simulink model "APP_SelSig1"  (R2016b)
settings: configuration reference "CodeGenConfigSet" (kept outside this file)
values from neighbouring files (symbols this model uses):
  APP_duLimErrPos_C = Calibration.Parameter    [init_APP_SelSig.m]
  APP_uAPPDef_C = Calibration.Parameter    [init_APP_SelSig.m]
  APP_uRaw2Offset_C = Calibration.Parameter    [init_APP_SelSig.m]
  MoFAPP_dRawSigFac_C = Calibration.Parameter    [init_APP_SelSig.m]
undefined symbols (not defined in the file or in its folder): APP_SelSig_DT
libraries: CXLib x3
settings Model: Creator=lenovo  LastModifiedBy=bianxuyin
settings ConfigSetRef: SourceLocation=Base Workspace

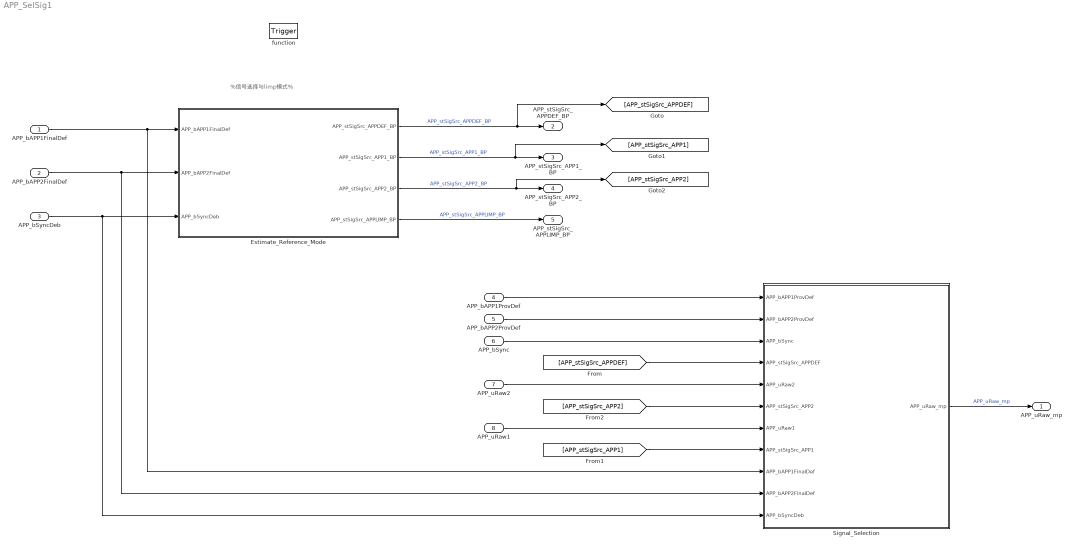
== system APP_SelSig1 ==
  note: %信号选择与limp模式%
  APP_bAPP1FinalDef : Inport  Description=Status Sensor 1 of the acceleration pedal finally defect  OutMin=0  OutMax=1  OutDataTypeStr=boolean
  APP_bAPP2FinalDef : Inport  Description=Status Sensor 2 of the acceleration pedal finally defect  Port=2  OutMin=0  OutMax=1  OutDataTypeStr=boolean
  APP_bSyncDeb : Inport  Description=Status debounced sync check  Port=3  OutMin=0  OutMax=1  OutDataTypeStr=boolean
  APP_bAPP1ProvDef : Inport  Description=Status Sensor 1 of the acceleration pedal temporary defect  Port=4  OutMin=0  OutMax=1  OutDataTypeStr=boolean
  APP_bAPP2ProvDef : Inport  Description=Status Sensor 2 of the acceleration pedal temporary defect  Port=5  OutMin=0  OutMax=1  OutDataTypeStr=boolean
  APP_bSync : Inport  Description=Status temporary sync check  Port=6  OutMin=0  OutMax=1  OutDataTypeStr=boolean
  APP_uRaw2 : Inport  Tag=mv  Description=Acceleration Pedal Position E  Port=7  OutMin=0  OutMax=5000  OutDataTypeStr=Ad_mv
  APP_uRaw1 : Inport  Tag=mv  Description=Acceleration Pedal Position D  Port=8  OutMin=0  OutMax=5000  OutDataTypeStr=Ad_mv
  function : TriggerPort  TriggerType=function-call  VariantControl=Variant
  Estimate_Reference_Mode : Subsystem
  Signal_Selection : Subsystem
  APP_uRaw_mp : Outport  Tag=mv  Description=Acceleration pedal position raw value  OutMin=0  OutMax=5000  OutDataTypeStr=Ad_mv
  APP_stSigSrc_APPDEF_BP : Outport  Description=both the sensors are defective. Use the default value  Port=2  OutMin=0  OutMax=1  OutDataTypeStr=boolean
  APP_stSigSrc_APP1_BP : Outport  Description=Sensor 1 is the reference variable, Sensor 2 value is defective  Port=3  OutMin=0  OutMax=1  OutDataTypeStr=boolean
  APP_stSigSrc_APP2_BP : Outport  Description=Sensor 2 is the reference variable,Sensor1 value is defective  Port=4  OutMin=0  OutMax=1  OutDataTypeStr=boolean
  APP_stSigSrc_APPLIMP_BP : Outport  Description=Substitute operation active, accelerator pedal sensor value and accelerator pedal sensor increase are limited  Port=5  OutMin=0  OutMax=1  OutDataTypeStr=boolean
  wires:
  Estimate_Reference_Mode/4(APP_stSigSrc_APPLIMP_BP) -> APP_stSigSrc_APPLIMP_BP/1  "APP_stSigSrc_APPLIMP_BP"
  Estimate_Reference_Mode/1(APP_stSigSrc_APPDEF_BP) -> [APP_stSigSrc_APPDEF], APP_stSigSrc_APPDEF_BP/1  "APP_stSigSrc_APPDEF_BP"
  Estimate_Reference_Mode/2(APP_stSigSrc_APP1_BP) -> [APP_stSigSrc_APP1], APP_stSigSrc_APP1_BP/1  "APP_stSigSrc_APP1_BP"
  Estimate_Reference_Mode/3(APP_stSigSrc_APP2_BP) -> APP_stSigSrc_APP2_BP/1, [APP_stSigSrc_APP2]  "APP_stSigSrc_APP2_BP"
  APP_bSyncDeb/1 -> Signal_Selection/11(APP_bSyncDeb), Estimate_Reference_Mode/3(APP_bSyncDeb)
  APP_bAPP2FinalDef/1 -> Signal_Selection/10(APP_bAPP2FinalDef), Estimate_Reference_Mode/2(APP_bAPP2FinalDef)
  APP_bAPP1FinalDef/1 -> Signal_Selection/9(APP_bAPP1FinalDef), Estimate_Reference_Mode/1(APP_bAPP1FinalDef)
  APP_bAPP1ProvDef/1 -> Signal_Selection/1(APP_bAPP1ProvDef)
  APP_bAPP2ProvDef/1 -> Signal_Selection/2(APP_bAPP2ProvDef)
  APP_bSync/1 -> Signal_Selection/3(APP_bSync)
  [APP_stSigSrc_APPDEF] -> Signal_Selection/4(APP_stSigSrc_APPDEF)
  APP_uRaw2/1 -> Signal_Selection/5(APP_uRaw2)
  [APP_stSigSrc_APP2] -> Signal_Selection/6(APP_stSigSrc_APP2)
  APP_uRaw1/1 -> Signal_Selection/7(APP_uRaw1)
  Signal_Selection/1(APP_uRaw_mp) -> APP_uRaw_mp/1  "APP_uRaw_mp"
  [APP_stSigSrc_APP1] -> Signal_Selection/8(APP_stSigSrc_APP1)

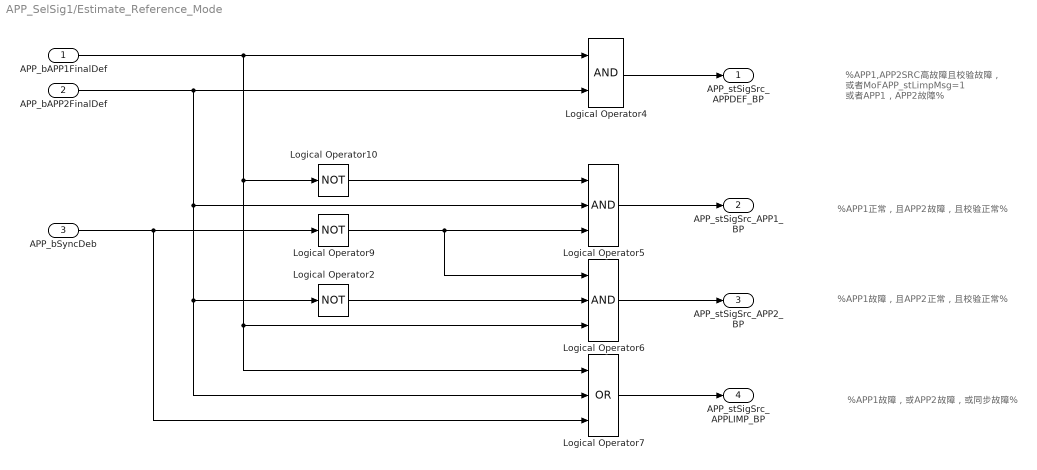
== system APP_SelSig1/Estimate_Reference_Mode ==
  note: %APP1正常，且APP2故障，且校验正常%
  note: %APP1故障，且APP2正常，且校验正常%
  note: %APP1故障，或APP2故障，或同步故障%
  note: %APP1,APP2SRC高故障且校验故障，
      | 或者MoFAPP_stLimpMsg=1
      | 或者APP1，APP2故障%
  APP_bAPP1FinalDef : Inport
  APP_bAPP2FinalDef : Inport  Port=2
  APP_bSyncDeb : Inport  Port=3
  Logical Operator10 : Logic  Operator=NOT  AllPortsSameDT=off  OutDataTypeStr=boolean
  Logical Operator2 : Logic  Operator=NOT  AllPortsSameDT=off  OutDataTypeStr=boolean
  Logical Operator4 : Logic  OutDataTypeStr=boolean
  Logical Operator5 : Logic  Inputs=3  OutDataTypeStr=boolean
  Logical Operator6 : Logic  Inputs=3  OutDataTypeStr=boolean
  Logical Operator7 : Logic  Operator=OR  Inputs=3  OutDataTypeStr=boolean
  Logical Operator9 : Logic  Operator=NOT  AllPortsSameDT=off  OutDataTypeStr=boolean
  APP_stSigSrc_APPDEF_BP : Outport
  APP_stSigSrc_APP1_BP : Outport  Port=2
  APP_stSigSrc_APP2_BP : Outport  Port=3
  APP_stSigSrc_APPLIMP_BP : Outport  Port=4
  wires:
  Logical Operator2/1 -> Logical Operator6/2
  Logical Operator9/1 -> Logical Operator5/3, Logical Operator6/1
  Logical Operator10/1 -> Logical Operator5/1
  APP_bSyncDeb/1 -> Logical Operator9/1, Logical Operator7/3
  APP_bAPP2FinalDef/1 -> Logical Operator4/2, Logical Operator7/2, Logical Operator2/1, Logical Operator5/2
  APP_bAPP1FinalDef/1 -> Logical Operator4/1, Logical Operator10/1, Logical Operator7/1, Logical Operator6/3
  Logical Operator7/1 -> APP_stSigSrc_APPLIMP_BP/1
  Logical Operator6/1 -> APP_stSigSrc_APP2_BP/1
  Logical Operator5/1 -> APP_stSigSrc_APP1_BP/1
  Logical Operator4/1 -> APP_stSigSrc_APPDEF_BP/1

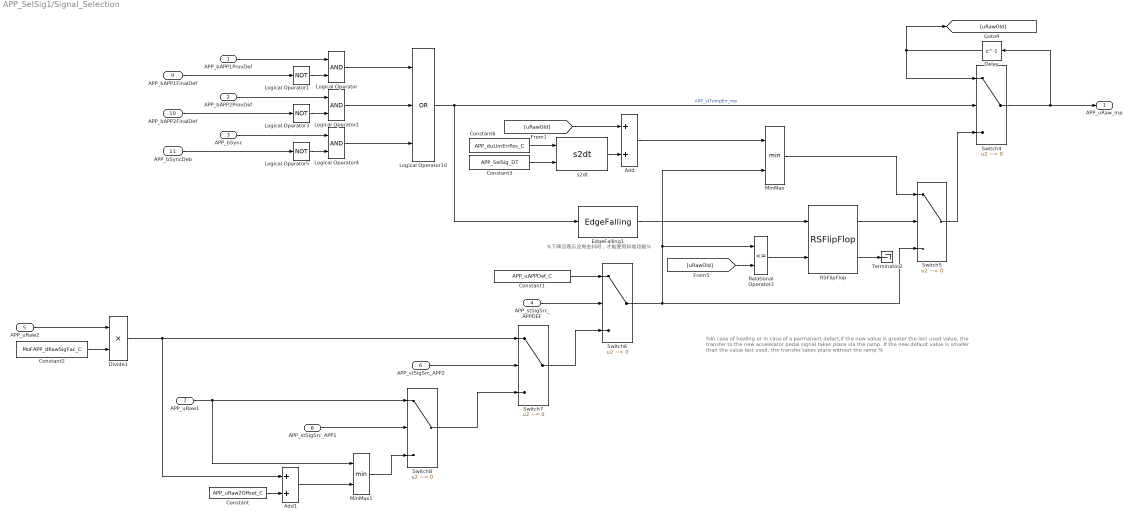
== system APP_SelSig1/Signal_Selection ==
  note: %下降沿表示没有去抖时，才能使用斜坡功能%
  note: %In case of healing or in case of a permanent defect,if the new value is greater the last used value,
      | the transfer to the new accelerator pedal signal takes place via the ramp. If the new default value
      | is smaller than the value last used, the transfer takes place without the ramp %
  APP_bAPP1ProvDef : Inport  Tag=-  Description=Status Sensor 1 of the acceleration pedal temporary defect  OutMin=0  OutMax=1  OutDataTypeStr=boolean
  APP_bAPP2ProvDef : Inport  Tag=-  Description=Status Sensor 2 of the acceleration pedal temporary defect  Port=2  OutMin=0  OutMax=1  OutDataTypeStr=boolean
  APP_bSync : Inport  Tag=-  Description=Status temporary sync check  Port=3  OutMin=0  OutMax=1  OutDataTypeStr=boolean
  APP_stSigSrc_APPDEF : Inport  Port=4
  APP_uRaw2 : Inport  Tag=mv  Description=Acceleration Pedal Position E  Port=5  OutMin=0  OutMax=5000  OutDataTypeStr=Ad_mv
  APP_stSigSrc_APP2 : Inport  Port=6
  APP_uRaw1 : Inport  Tag=mv  Description=Acceleration Pedal Position D  Port=7  OutMin=0  OutMax=5000  OutDataTypeStr=Ad_mv
  APP_stSigSrc_APP1 : Inport  Port=8
  APP_bAPP1FinalDef : Inport  Port=9
  APP_bAPP2FinalDef : Inport  Port=10
  APP_bSyncDeb : Inport  Port=11
  Add : Sum
  Add1 : Sum  InputSameDT=on
  Constant : Constant  RequirementInfo={'other' 'APP_requirements.doc' '@Simulink_requirement_item_21' 'true' '信号输出' '' } %GIDa_518cb01d_b25b_4388_a648_8c80e3d174e0  Value=APP_uRaw2Offset_C
  Constant1 : Constant  RequirementInfo={'other' 'APP_requirements.doc' '@Simulink_requirement_item_21' 'true' '信号输出' '' } %GIDa_55cd5498_cb96_4c81_8024_1b86d120cf7e  Value=APP_uAPPDef_C
  Constant2 : Constant  Value=MoFAPP_dRawSigFac_C  SampleTime=-1
  Constant3 : Constant  Value=APP_SelSig_DT  OutDataTypeStr=Inherit: Inherit via back propagation
  Constant6 : Constant  Value=APP_duLimErrPos_C
  Delay : Delay  DelayLength=1  InitialCondition=0
  Divide1 : Product  Inputs=**  OutDataTypeStr=Ad_mv
  EdgeFalling1 : CXLib/EdgeFalling  RequirementInfo={'other' 'APP_requirements.doc' '@Simulink_requirement_item_21' 'true' '信号输出' '' } %GIDa_4288bea6_2219_4ace_9b7e_63daecb36290
  Logical Operator : Logic  OutDataTypeStr=boolean
  Logical Operator1 : Logic  Operator=NOT  AllPortsSameDT=off  OutDataTypeStr=boolean
  Logical Operator10 : Logic  RequirementInfo={'other' 'APP_requirements.doc' '@Simulink_requirement_item_21' 'true' '信号输出' '' } %GIDa_c9f968ec_7aa3_41a8_9cc9_f89bf0f53934  Operator=OR  Inputs=3  OutDataTypeStr=boolean
  Logical Operator2 : Logic  OutDataTypeStr=boolean
  Logical Operator3 : Logic  Operator=NOT  AllPortsSameDT=off  OutDataTypeStr=boolean
  Logical Operator4 : Logic  OutDataTypeStr=boolean
  Logical Operator5 : Logic  Operator=NOT  AllPortsSameDT=off  OutDataTypeStr=boolean
  MinMax : MinMax  Inputs=2
  MinMax1 : MinMax  Inputs=2  InputSameDT=on
  RSFlipFlop : CXLib/RSFlipFlop  RequirementInfo={'other' 'APP_requirements.doc' '@Simulink_requirement_item_21' 'true' '信号输出' '' } %GIDa_2a0c15bf_1d67_41a3_a610_23d56195d123
  Relational Operator3 : RelationalOperator  RequirementInfo={'other' 'APP_requirements.doc' '@Simulink_requirement_item_21' 'true' '信号输出' '' } %GIDa_dd8df7f8_f262_4ae1_8fb8_d87d478286bb  Operator=<=  OutDataTypeStr=boolean  RndMeth=Nearest  InputSameDT=on
  Switch4 : Switch  RequirementInfo={'other' 'APP_requirements.doc' '@Simulink_requirement_item_21' 'true' '信号输出' '' } %GIDa_c9f01514_bebf_41fe_82d8_fe6fe3749094  Criteria=u2 ~= 0  InputSameDT=on
  Switch5 : Switch  RequirementInfo={'other' 'APP_requirements.doc' '@Simulink_requirement_item_21' 'true' '信号输出' '' } %GIDa_750b240f_9d38_4078_a4a7_5f2976992d4a  Criteria=u2 ~= 0  InputSameDT=on
  Switch6 : Switch  RequirementInfo={'other' 'APP_requirements.doc' '@Simulink_requirement_item_21' 'true' '信号输出' '' } %GIDa_4e4fa6a0_d5c7_4234_b382_721fdb48599f  Criteria=u2 ~= 0  InputSameDT=on
  Switch7 : Switch  RequirementInfo={'other' 'APP_requirements.doc' '@Simulink_requirement_item_21' 'true' '信号输出' '' } %GIDa_1c425b2d_5403_4593_8968_9a1285cfe668  Criteria=u2 ~= 0  InputSameDT=on
  Switch8 : Switch  RequirementInfo={'other' 'APP_requirements.doc' '@Simulink_requirement_item_21' 'true' '信号输出' '' } %GIDa_da73960f_2146_479d_a442_0600f38916ee  Criteria=u2 ~= 0  InputSameDT=on
  Terminator2 : Terminator
  s2dt : CXLib/s2dt
  APP_uRaw_mp : Outport  Tag=mv  Description=Acceleration pedal position raw value  OutMin=0  OutMax=5000  OutDataTypeStr=Ad_mv
  wires:
  APP_bAPP1FinalDef/1 -> Logical Operator1/1
  APP_bAPP2FinalDef/1 -> Logical Operator3/1
  APP_bSyncDeb/1 -> Logical Operator5/1
  Divide1/1 -> Switch7/1, Add1/1
  Constant/1 -> Add1/2
  APP_uRaw1/1 -> Switch8/1, MinMax1/1
  APP_stSigSrc_APP2/1 -> Switch7/2
  Switch8/1 -> Switch7/3
  APP_uRaw2/1 -> Divide1/1
  Constant1/1 -> Switch6/1
  Add1/1 -> MinMax1/2
  APP_stSigSrc_APP1/1 -> Switch8/2
  APP_stSigSrc_APPDEF/1 -> Switch6/2
  MinMax1/1 -> Switch8/3
  Switch7/1 -> Switch6/3
  Constant2/1 -> Divide1/2
  EdgeFalling1/1 -> RSFlipFlop/1
  Relational Operator3/1 -> RSFlipFlop/2
  Switch4/1 -> APP_uRaw_mp/1, Delay/1
  Delay/1 -> Switch4/1, [uRawOld]
  RSFlipFlop/1 -> Switch5/2
  Switch5/1 -> Switch4/3
  RSFlipFlop/2 -> Terminator2/1
  Logical Operator10/1 -> Switch4/2, EdgeFalling1/1  "APP_stTempErr_mp"
  APP_bAPP1ProvDef/1 -> Logical Operator/1
  Logical Operator1/1 -> Logical Operator/2
  APP_bAPP2ProvDef/1 -> Logical Operator2/1
  Logical Operator3/1 -> Logical Operator2/2
  Logical Operator5/1 -> Logical Operator4/2
  Logical Operator/1 -> Logical Operator10/1
  Logical Operator2/1 -> Logical Operator10/2
  Logical Operator4/1 -> Logical Operator10/3
  APP_bSync/1 -> Logical Operator4/1
  [uRawOld] -> Relational Operator3/2
  Switch6/1 -> Switch5/3, Relational Operator3/1, MinMax/2
  [uRawOld] -> Add/1
  Add/1 -> MinMax/1
  MinMax/1 -> Switch5/1
  s2dt/1 -> Add/2
  Constant6/1 -> s2dt/1
  Constant3/1 -> s2dt/2
